simulink model "rosio"  (R2015a)
settings: Solver=ode3  StartTime=0.0  StopTime=inf  FixedStep=0.01  RelTol=1e-3
libraries: robotlib x2
settings Model: Creator=corkep  LastModifiedBy=corkep

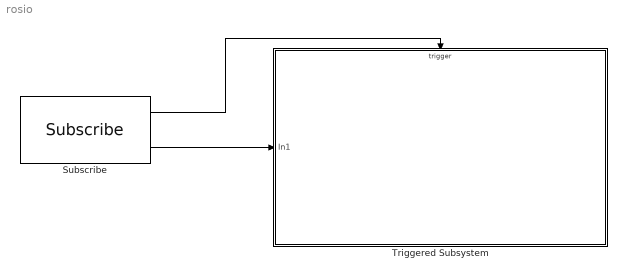
== system rosio ==
  Subscribe : robotlib/Subscribe  SourceLibraryInfo=This block requires Robotics System Toolbox  topicSource=Specify your own  topic=/MyTopic2  messageType=std_msgs/String  sampleTime=-1  messageQueueLength=1
  Triggered Subsystem : Subsystem  TreatAsAtomicUnit=on
  wires:
  Subscribe/2 -> Triggered Subsystem/1(In1)
  Subscribe/1 -> Triggered Subsystem/Trigger

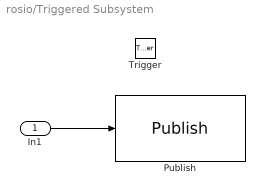
== system rosio/Triggered Subsystem ==
  In1 : Inport
  Trigger : TriggerPort
  Publish : robotlib/Publish  SourceLibraryInfo=This block requires Robotics System Toolbox  topicSource=Specify your own  topic=/MyTopic  messageType=std_msgs/String  messageQueueLength=1
  wires:
  In1/1 -> Publish/1
